simulink model "REXduino_masks"  (Simulink 3.00)
settings: Solver=ode45  SolverMode=SingleTasking  StartTime=0.0  StopTime=10.0  RelTol=1e-3
libraries: logiclib x194, mathlib x116, analoglib x15, genlib x12, speclib x4
(part 1 of 2)
settings Model: ExtModeTrigMode=normal  ExtModeArmWhenConnect=on  Creator=jsobota  LastModifiedBy=XPMUser

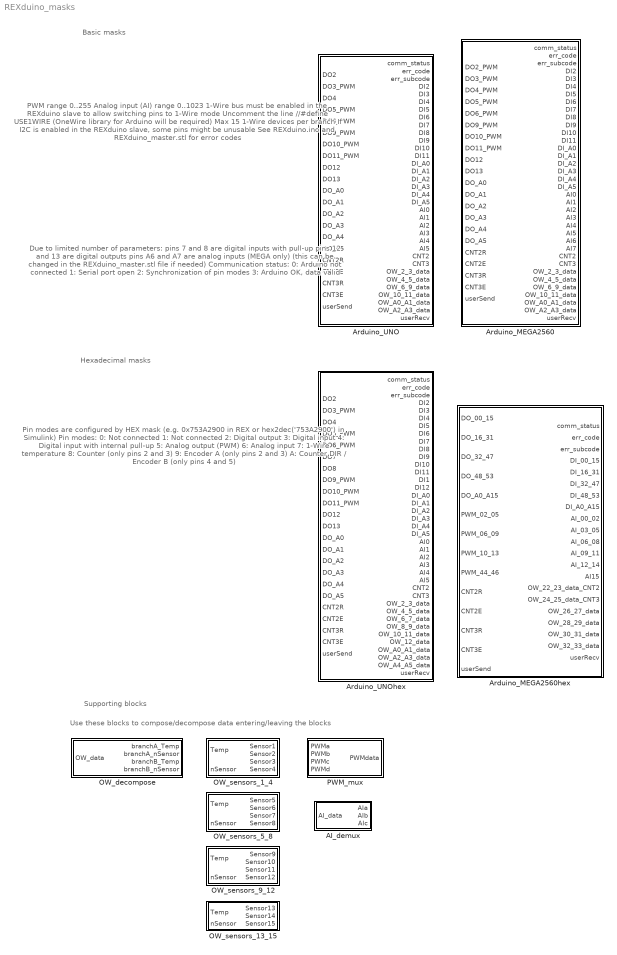
== system REXduino_masks ==
  note: Basic masks
  note: PWM range 0..255
      |
      | Analog input (AI) range 0..1023
      |
      | 1-Wire bus must be enabled in the REXduino slave
      | to allow switching pins to 1-Wire mode
      | Uncomment the line //#define USE1WIRE
      | (OneWire library for Arduino will be required)
      |
      | Max 15 1-Wire devices per branch
      |
      | If I2C is enabled in the REXduino slave, some pins
      | might be unusable
      |
      | See REXduino.ino and REXduino_master.stl for error codes
  note: Hexadecimal masks
  note: Pin modes are configured by HEX mask
      |    (e.g. 0x753A2900 in REX or hex2dec('753A2900') in Simulink)
      |
      | Pin modes:
      | 0: Not connected
      | 1: Not connected
      | 2: Digital output
      | 3: Digital input
      | 4: Digital input with internal pull-up
      | 5: Analog output (PWM)
      | 6: Analog input
      | 7: 1-Wire temperature
      | 8: Counter (only pins 2 and 3)
      | 9: Encoder A (only pins 2 and 3)
      | A: Counter DIR / Encoder B (only pins 4 and 5)
  note: Supporting blocks
  note: Use these blocks to compose/decompose data entering/leaving the blocks
  note: Due to limited number of parameters:
      | pins 7 and 8 are digital inputs with pull-up
      | pins 12 and 13 are digital outputs
      | pins A6 and A7 are analog inputs (MEGA only)
      | (this can be changed in the REXduino_master.stl file if needed)
      |
      | Communication status:
      | 0: Arduino not connected
      | 1: Serial port open
      | 2: Synchronization of pin modes
      | 3: Arduino OK, data valid
  AI_demux : Subsystem
      mask Type: REX sequence
  Arduino_MEGA2560 : Subsystem  mask(REX sequence){comPort=/dev/ttyACM0, pinmode2=1: Not connected, pinmode3=1: Not connected, pinmode4=1: Not connected, pinmode5=1: Not connected, pinmode6=1: Not connected, pinmode9=1: Not connected, pinmode10=1: Not connected, pinmode11=1: Not connected, pinmodeA0=1: Not connected, pinmodeA1=1: Not connected, pinmodeA2=1: Not connected, pinmodeA3=1: Not connected, pinmodeA4=1: Not connected, pinmodeA5=1: Not connected}
      mask prompts: comPort "Serial device, e.g. COM7, /dev/ttyACM0, /dev/ttyUSB0 etc."; pinmode2 "Pin 2 mode"; pinmode3 "Pin 2 mode"; pinmode4 "Pin 2 mode"; pinmode5 "Pin 2 mode"; pinmode6 "Pin 2 mode"; pinmode9 "Pin 2 mode"; pinmode10 "Pin 2 mode"; pinmode11 "Pin 2 mode"; pinmodeA0 "Pin 2 mode"; pinmodeA1 "Pin 2 mode"; pinmodeA2 "Pin 2 mode"; pinmodeA3 "Pin 2 mode"; pinmodeA4 "Pin 2 mode"; pinmodeA5 "Pin 2 mode"
      mask StyleString: edit,popup(1: Not connected|2: Digital output|3: Digital input|4: Digital input with internal pull-up|5: PWM (analog output)|6: --- N/A for this pin ---|7: 1-Wire temperature|8: Counter|9: Encoder),popup(1: Not connected|2: Digital output|3: Digital input|4: Digital input with internal pull-up|5: PWM (analog output)|6: --- N/A for this pin ---|7: 1-Wire temperature|8: Counter|9: Encoder),popup(1: Not connected|2: Digital output|3: Digital input|4: Digital input with internal pull-up|5: PWM (analog output)|6: --- N/A for this pin ---|7: 1-Wire temperature|8: --- N/A for this pin ---|9: --- N/A for this pin ---|10: Counter DIR / Encoder B),popup(1: Not connected|2: Digital output|3: Digital input|4: Digital input with internal pull-up|5: PWM (analog output)|6: --- N/A for this pin ---|7: 1-Wire temperature|8: --- N/A for this pin ---|9: --- N/A for this pin ---|10: Counter DIR / Encoder B),popup(1: Not connected|2: Digital output|3: Digital input|4: Digital input with internal pull-up|5: PWM (analog output)|6: --- N/A for this pin ---|7: 1-Wire temperature),popup(1: Not connected|2: Digital output|3: Digital input|4: Digital input with internal pull-up|5: PWM (analog output)|6: --- N/A for this pin ---|7: 1-Wire temperature),popup(1: Not connected|2: Digital output|3: Digital input|4: Digital input with internal pull-up|5: PWM (analog output)|6: --- N/A for this pin ---|7: 1-Wire temperature),popup(1: Not connected|2: Digital output|3: Digital input|4: Digital input with internal pull-up|5: PWM (analog output)|6: --- N/A for this pin|7: 1-Wire temperature),popup(1: Not connected|2: Digital output|3: Digital input|4: Digital input with internal pull-up|5: --- N/A for this pin ---|6: Analog input|7: 1-Wire temperature),popup(1: Not connected|2: Digital output|3: Digital input|4: Digital input with internal pull-up|5: --- N/A for this pin ---|6: Analog input|7: 1-Wire temperature),popup(1: Not connected|2: Digital output|3: Digital input|4: Digital input with internal pull-up|5: --- N/A for this pin ---|6: Analog input|7: 1-Wire temperature),popup(1: Not connected|2: Digital output|3: Digital input|4: Digital input with internal pull-up|5: --- N/A for this pin ---|6: Analog input|7: 1-Wire temperature),popup(1: Not connected|2: Digital output|3: Digital input|4: Digital input with internal pull-up|5: --- N/A for this pin ---|6: Analog input|7: 1-Wire temperature),popup(1: Not connected|2: Digital output|3: Digital input|4: Digital input with internal pull-up|5: --- N/A for this pin ---|6: Analog input|7: 1-Wire temperature)
      mask CallbackString:
      | REXduino_mask_comPortNo = get_param(gcb,'comPort');
      | REXduino_mask_comPortNo = sscanf(fliplr(REXduino_mask_comPortNo),'%u',1);
      | if ( ~isempty(REXduino_mask_comPortNo) & (REXduino_mask_comPortNo<100) )
      | set_param([gcb '/CNI_comPortNo'],'icn',fliplr(num2str(REXduino_mask_comPortNo)))
      | else
      | set_param([gcb '/CNI_comPortNo'],'icn','15')
      | end
      | clear REXduino_mask_comPortNo||||||||||||||
  Arduino_MEGA2560hex : Subsystem  mask(REX sequence){comPort=/dev/ttyACM0, pinmodes_00_07=0, pinmodes_08_15=0, pinmodes_16_23=0, pinmodes_24_31=0, pinmodes_32_39=0, pinmodes_40_47=0, pinmodes_48_53=0, pinmodes_A0_A7=0, pinmodes_A8_A15=0}
      mask prompts: comPort "Serial device, e.g. COM7, /dev/ttyACM0, /dev/ttyUSB0 etc."; pinmodes_00_07 "Pin modes 0 to 7 (0 and 1 ignored)"; pinmodes_08_15 "Pin modes 8 to 15"; pinmodes_16_23 "Pin modes 16 to 23"; pinmodes_24_31 "Pin modes 24 to 31"; pinmodes_32_39 "Pin modes 32 to 39"; pinmodes_40_47 "Pin modes 40 to 47"; pinmodes_48_53 "Pin modes 48 to 53"; pinmodes_A0_A7 "Pin modes A0 to A7"; pinmodes_A8_A15 "Pin modes A8 to A15"
      mask CallbackString:
      | REXduino_mask_comPortNo = get_param(gcb,'comPort');
      | REXduino_mask_comPortNo = sscanf(fliplr(REXduino_mask_comPortNo),'%u',1);
      | if ( ~isempty(REXduino_mask_comPortNo) & (REXduino_mask_comPortNo<100) )
      | set_param([gcb '/CNI_comPortNo'],'icn',fliplr(num2str(REXduino_mask_comPortNo)))
      | else
      | set_param([gcb '/CNI_comPortNo'],'icn','15')
      | end
      | clear REXduino_mask_comPortNo|||||||||
  Arduino_UNO : Subsystem  mask(REX sequence){comPort=/dev/ttyACM0, pinmode2=1: Not connected, pinmode3=1: Not connected, pinmode4=1: Not connected, pinmode5=1: Not connected, pinmode6=1: Not connected, pinmode9=1: Not connected, pinmode10=1: Not connected, pinmode11=1: Not connected, pinmodeA0=1: Not connected, pinmodeA1=1: Not connected, pinmodeA2=1: Not connected, pinmodeA3=1: Not connected, pinmodeA4=1: Not connected, pinmodeA5=1: Not connected}
      mask prompts: comPort "Serial device, e.g. COM7, /dev/ttyACM0, /dev/ttyUSB0 etc."; pinmode2 "Pin 2 mode"; pinmode3 "Pin 2 mode"; pinmode4 "Pin 2 mode"; pinmode5 "Pin 2 mode"; pinmode6 "Pin 2 mode"; pinmode9 "Pin 2 mode"; pinmode10 "Pin 2 mode"; pinmode11 "Pin 2 mode"; pinmodeA0 "Pin 2 mode"; pinmodeA1 "Pin 2 mode"; pinmodeA2 "Pin 2 mode"; pinmodeA3 "Pin 2 mode"; pinmodeA4 "Pin 2 mode"; pinmodeA5 "Pin 2 mode"
      mask StyleString: edit,popup(1: Not connected|2: Digital output|3: Digital input|4: Digital input with internal pull-up|5: --- N/A for this pin ---|6: --- N/A for this pin ---|7: 1-Wire temperature|8: Counter|9: Encoder A),popup(1: Not connected|2: Digital output|3: Digital input|4: Digital input with internal pull-up|5: PWM (analog output)|6: --- N/A for this pin ---|7: 1-Wire temperature|8: Counter|9: Encoder A),popup(1: Not connected|2: Digital output|3: Digital input|4: Digital input with internal pull-up|5: --- N/A for this pin ---|6: --- N/A for this pin ---|7: 1-Wire temperature|8: --- N/A for this pin ---|9: --- N/A for this pin ---|10: Counter DIR / Encoder B),popup(1: Not connected|2: Digital output|3: Digital input|4: Digital input with internal pull-up|5: PWM (analog output)|6: --- N/A for this pin ---|7: 1-Wire temperature|8: --- N/A for this pin ---|9: --- N/A for this pin ---|10: Counter DIR / Encoder B),popup(1: Not connected|2: Digital output|3: Digital input|4: Digital input with internal pull-up|5: PWM (analog output)|6: --- N/A for this pin ---|7: 1-Wire temperature),popup(1: Not connected|2: Digital output|3: Digital input|4: Digital input with internal pull-up|5: PWM (analog output)|6: --- N/A for this pin ---|7: 1-Wire temperature),popup(1: Not connected|2: Digital output|3: Digital input|4: Digital input with internal pull-up|5: PWM (analog output)|6: --- N/A for this pin ---|7: 1-Wire temperature),popup(1: Not connected|2: Digital output|3: Digital input|4: Digital input with internal pull-up|5: PWM (analog output)|6: --- N/A for this pin ---|7: 1-Wire temperature),popup(1: Not connected|2: Digital output|3: Digital input|4: Digital input with internal pull-up|5: --- N/A for this pin ---|6: Analog input|7: 1-Wire temperature),popup(1: Not connected|2: Digital output|3: Digital input|4: Digital input with internal pull-up|5: --- N/A for this pin ---|6: Analog input|7: 1-Wire temperature),popup(1: Not connected|2: Digital output|3: Digital input|4: Digital input with internal pull-up|5: --- N/A for this pin ---|6: Analog input|7: 1-Wire temperature),popup(1: Not connected|2: Digital output|3: Digital input|4: Digital input with internal pull-up|5: --- N/A for this pin ---|6: Analog input|7: 1-Wire temperature),popup(1: Not connected|2: Digital output|3: Digital input|4: Digital input with internal pull-up|5: --- N/A for this pin ---|6: Analog input|7: 1-Wire temperature),popup(1: Not connected|2: Digital output|3: Digital input|4: Digital input with internal pull-up|5: --- N/A for this pin ---|6: Analog input|7: 1-Wire temperature)
      mask CallbackString:
      | REXduino_mask_comPortNo = get_param(gcb,'comPort');
      | REXduino_mask_comPortNo = sscanf(fliplr(REXduino_mask_comPortNo),'%u',1);
      | if ( ~isempty(REXduino_mask_comPortNo) & (REXduino_mask_comPortNo<100) )
      | set_param([gcb '/CNI_comPortNo'],'icn',fliplr(num2str(REXduino_mask_comPortNo)))
      | else
      | set_param([gcb '/CNI_comPortNo'],'icn','15')
      | end
      | clear REXduino_mask_comPortNo||||||||||||||
  Arduino_UNOhex : Subsystem  mask(REX sequence){comPort=/dev/ttyACM0, pinmodes_00_07=0, pinmodes_08_13=0, pinmodes_A0_A5=0}
      mask prompts: comPort "Serial device, e.g. COM7, /dev/ttyACM0, /dev/ttyUSB0 etc."; pinmodes_00_07 "Pin modes 0 to 7 (0 and 1 ignored)"; pinmodes_08_13 "Pin modes 8 to 13"; pinmodes_A0_A5 "Pin modes A0 to A5"
      mask CallbackString:
      | REXduino_mask_comPortNo = get_param(gcb,'comPort');
      | REXduino_mask_comPortNo = sscanf(fliplr(REXduino_mask_comPortNo),'%u',1);
      | if ( ~isempty(REXduino_mask_comPortNo) & (REXduino_mask_comPortNo<100) )
      | set_param([gcb '/CNI_comPortNo'],'icn',fliplr(num2str(REXduino_mask_comPortNo)))
      | else
      | set_param([gcb '/CNI_comPortNo'],'icn','15')
      | end
      | clear REXduino_mask_comPortNo|||
  OW_decompose : Subsystem
      mask Type: REX sequence
  OW_sensors_13_15 : Subsystem
      mask Type: REX sequence
  OW_sensors_1_4 : Subsystem
      mask Type: REX sequence
  OW_sensors_5_8 : Subsystem
      mask Type: REX sequence
  OW_sensors_9_12 : Subsystem
      mask Type: REX sequence
  PWM_mux : Subsystem
      mask Type: REX sequence

== system REXduino_masks/AI_demux ==
  AI_data : Inport  Port=1  PortWidth=-1  SampleTime=-1  DataType=auto
      settings: SignalType=auto
  BITOP_1 : logiclib/BITOP  iop=6: Shift Right
  BITOP_10 : logiclib/BITOP  iop=3: Bit AND
  BITOP_2 : logiclib/BITOP  iop=3: Bit AND
  BITOP_3 : logiclib/BITOP  iop=6: Shift Right
  BITOP_4 : logiclib/BITOP  iop=3: Bit AND
  CNI : mathlib/CNI  icn=1023
  CNI_1 : mathlib/CNI  icn=10
  AIa : Outport  Port=1
  AIb : Outport  Port=2
  AIc : Outport  Port=3
  wires:
  AI_data/1 -> BITOP_1/1, BITOP_10/1
  BITOP_1/1 -> BITOP_2/1, BITOP_3/1
  BITOP_10/1 -> AIa/1
  BITOP_2/1 -> AIb/1
  BITOP_3/1 -> BITOP_4/1
  BITOP_4/1 -> AIc/1
  CNI/1 -> BITOP_10/2, BITOP_2/2, BITOP_4/2
  CNI_1/1 -> BITOP_1/2, BITOP_3/2

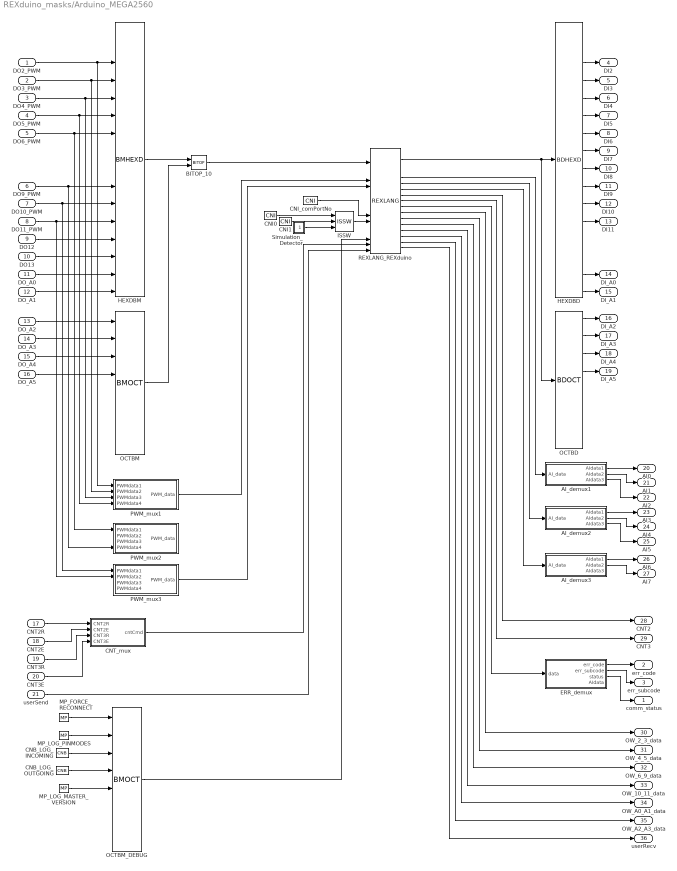
== system REXduino_masks/Arduino_MEGA2560 ==
  DO2_PWM : Inport  Port=1  PortWidth=-1  SampleTime=-1  DataType=auto
      settings: SignalType=auto
  DO3_PWM : Inport  Port=2  PortWidth=-1  SampleTime=-1  DataType=auto
      settings: SignalType=auto
  DO4_PWM : Inport  Port=3  PortWidth=-1  SampleTime=-1  DataType=auto
      settings: SignalType=auto
  DO5_PWM : Inport  Port=4  PortWidth=-1  SampleTime=-1  DataType=auto
      settings: SignalType=auto
  DO6_PWM : Inport  Port=5  PortWidth=-1  SampleTime=-1  DataType=auto
      settings: SignalType=auto
  DO9_PWM : Inport  Port=6  PortWidth=-1  SampleTime=-1  DataType=auto
      settings: SignalType=auto
  DO10_PWM : Inport  Port=7  PortWidth=-1  SampleTime=-1  DataType=auto
      settings: SignalType=auto
  DO11_PWM : Inport  Port=8  PortWidth=-1  SampleTime=-1  DataType=auto
      settings: SignalType=auto
  DO12 : Inport  Port=9  PortWidth=-1  SampleTime=-1  DataType=auto
      settings: SignalType=auto
  DO13 : Inport  Port=10  PortWidth=-1  SampleTime=-1  DataType=auto
      settings: SignalType=auto
  DO_A0 : Inport  Port=11  PortWidth=-1  SampleTime=-1  DataType=auto
      settings: SignalType=auto
  DO_A1 : Inport  Port=12  PortWidth=-1  SampleTime=-1  DataType=auto
      settings: SignalType=auto
  DO_A2 : Inport  Port=13  PortWidth=-1  SampleTime=-1  DataType=auto
      settings: SignalType=auto
  DO_A3 : Inport  Port=14  PortWidth=-1  SampleTime=-1  DataType=auto
      settings: SignalType=auto
  DO_A4 : Inport  Port=15  PortWidth=-1  SampleTime=-1  DataType=auto
      settings: SignalType=auto
  DO_A5 : Inport  Port=16  PortWidth=-1  SampleTime=-1  DataType=auto
      settings: SignalType=auto
  CNT2R : Inport  Port=17  PortWidth=-1  SampleTime=-1  DataType=auto
      settings: SignalType=auto
  CNT2E : Inport  Port=18  PortWidth=-1  SampleTime=-1  DataType=auto
      settings: SignalType=auto
  CNT3R : Inport  Port=19  PortWidth=-1  SampleTime=-1  DataType=auto
      settings: SignalType=auto
  CNT3E : Inport  Port=20  PortWidth=-1  SampleTime=-1  DataType=auto
      settings: SignalType=auto
  userSend : Inport  Port=21  PortWidth=-1  SampleTime=-1  DataType=auto
      settings: SignalType=auto
  AI_demux1 : Subsystem
      mask Type: REX sequence
  AI_demux2 : Subsystem
      mask Type: REX sequence
  AI_demux3 : Subsystem
      mask Type: REX sequence
  BITOP_10 : logiclib/BITOP  iop=2: Bit OR
  CNB_LOG_INCOMING : mathlib/CNB  YCN=off
  CNB_LOG_OUTGOING : mathlib/CNB  YCN=off
  CNI0 : mathlib/CNI  icn=0
  CNI1 : mathlib/CNI  icn=1
  CNI_comPortNo : mathlib/CNI  icn=15
  CNT_mux : Subsystem
      mask Type: REX sequence
  ERR_demux : Subsystem
      mask Type: REX sequence
  HEXDBD : logiclib/BDHEXD  shift=0
  HEXDBM : logiclib/BMHEXD  shift=0
  ISSW : logiclib/ISSW
  MP_FORCE_RECONNECT : genlib/MP  pwidth=10  BSTATE=off  RPTF=off
  MP_LOG_MASTER_VERSION : genlib/MP  pwidth=10  BSTATE=off  RPTF=off
  MP_LOG_PINMODES : genlib/MP  pwidth=10  BSTATE=off  RPTF=off
  OCTBD : logiclib/BDOCT  shift=16
  OCTBM : logiclib/BMOCT  shift=16
  OCTBM_DEBUG : logiclib/BMOCT  shift=0
  PWM_mux1 : Subsystem
      mask Type: REX sequence
  PWM_mux2 : Subsystem
      mask Type: REX sequence
  PWM_mux3 : Subsystem
      mask Type: REX sequence
  REXLANG_REXduino : speclib/REXLANG  strs=0  tab_matlab=MORE  srcname=REXduino_master.c  srctype=1: C-like  stack=0  debug=1: No check  p0=comPort  p1=pinmode2  p2=pinmode3  p3=pinmode4  p4=pinmode5  p5=pinmode6  p6=pinmode9  p7=pinmode10  p8=pinmode11  p9=pinmodeA0  p10=pinmodeA1  p11=pinmodeA2  p12=pinmodeA3  p13=pinmodeA4  p14=pinmodeA5  p15=3
  Simulation_Detector : Subsystem
      mask Type: REX sequence
  comm_status : Outport  Port=1
  err_code : Outport  Port=2
  err_subcode : Outport  Port=3
  DI2 : Outport  Port=4
  DI3 : Outport  Port=5
  DI4 : Outport  Port=6
  DI5 : Outport  Port=7
  DI6 : Outport  Port=8
  DI7 : Outport  Port=9
  DI8 : Outport  Port=10
  DI9 : Outport  Port=11
  DI10 : Outport  Port=12
  DI11 : Outport  Port=13
  DI_A0 : Outport  Port=14
  DI_A1 : Outport  Port=15
  DI_A2 : Outport  Port=16
  DI_A3 : Outport  Port=17
  DI_A4 : Outport  Port=18
  DI_A5 : Outport  Port=19
  AI0 : Outport  Port=20
  AI1 : Outport  Port=21
  AI2 : Outport  Port=22
  AI3 : Outport  Port=23
  AI4 : Outport  Port=24
  AI5 : Outport  Port=25
  AI6 : Outport  Port=26
  AI7 : Outport  Port=27
  CNT2 : Outport  Port=28
  CNT3 : Outport  Port=29
  OW_2_3_data : Outport  Port=30
  OW_4_5_data : Outport  Port=31
  OW_6_9_data : Outport  Port=32
  OW_10_11_data : Outport  Port=33
  OW_A0_A1_data : Outport  Port=34
  OW_A2_A3_data : Outport  Port=35
  userRecv : Outport  Port=36
  wires:
  AI_demux1/1(AIdata1) -> AI0/1
  AI_demux1/2(AIdata2) -> AI1/1
  AI_demux1/3(AIdata3) -> AI2/1
  AI_demux2/1(AIdata1) -> AI3/1
  AI_demux2/2(AIdata2) -> AI4/1
  AI_demux2/3(AIdata3) -> AI5/1
  AI_demux3/1(AIdata1) -> AI6/1
  AI_demux3/2(AIdata2) -> AI7/1
  BITOP_10/1 -> REXLANG_REXduino/3
  CNB_LOG_INCOMING/1 -> OCTBM_DEBUG/3
  CNB_LOG_OUTGOING/1 -> OCTBM_DEBUG/4
  CNI0/1 -> ISSW/1
  CNI1/1 -> ISSW/2
  CNI_comPortNo/1 -> REXLANG_REXduino/12
  CNT2E/1 -> CNT_mux/2(CNT2E)
  CNT2R/1 -> CNT_mux/1(CNT2R)
  CNT3E/1 -> CNT_mux/4(CNT3E)
  CNT3R/1 -> CNT_mux/3(CNT3R)
  CNT_mux/1(cntCmd) -> REXLANG_REXduino/17
  DO10_PWM/1 -> HEXDBM/11, PWM_mux3/1(PWMdata1)
  DO11_PWM/1 -> HEXDBM/12, PWM_mux3/2(PWMdata2)
  DO12/1 -> HEXDBM/13
  DO13/1 -> HEXDBM/14
  DO2_PWM/1 -> HEXDBM/3, PWM_mux1/1(PWMdata1)
  DO3_PWM/1 -> HEXDBM/4, PWM_mux1/2(PWMdata2)
  DO4_PWM/1 -> HEXDBM/5, PWM_mux1/3(PWMdata3)
  DO5_PWM/1 -> HEXDBM/6, PWM_mux1/4(PWMdata4)
  DO6_PWM/1 -> HEXDBM/7, PWM_mux2/1(PWMdata1)
  DO9_PWM/1 -> HEXDBM/10, PWM_mux2/4(PWMdata4)
  DO_A0/1 -> HEXDBM/15
  DO_A1/1 -> HEXDBM/16
  DO_A2/1 -> OCTBM/1
  DO_A3/1 -> OCTBM/2
  DO_A4/1 -> OCTBM/3
  DO_A5/1 -> OCTBM/4
  ERR_demux/1(err_code) -> err_code/1
  ERR_demux/2(err_subcode) -> err_subcode/1
  ERR_demux/3(status) -> comm_status/1
  HEXDBD/3 -> DI2/1
  HEXDBD/4 -> DI3/1
  HEXDBD/5 -> DI4/1
  HEXDBD/6 -> DI5/1
  HEXDBD/7 -> DI6/1
  HEXDBD/8 -> DI7/1
  HEXDBD/9 -> DI8/1
  HEXDBD/10 -> DI9/1
  HEXDBD/11 -> DI10/1
  HEXDBD/12 -> DI11/1
  HEXDBD/15 -> DI_A0/1
  HEXDBD/16 -> DI_A1/1
  HEXDBM/1 -> BITOP_10/1
  ISSW/1 -> REXLANG_REXduino/13
  MP_FORCE_RECONNECT/1 -> OCTBM_DEBUG/1
  MP_LOG_MASTER_VERSION/1 -> OCTBM_DEBUG/5
  MP_LOG_PINMODES/1 -> OCTBM_DEBUG/2
  OCTBD/1 -> DI_A2/1
  OCTBD/2 -> DI_A3/1
  OCTBD/3 -> DI_A4/1
  OCTBD/4 -> DI_A5/1
  OCTBM/1 -> BITOP_10/2
  OCTBM_DEBUG/1 -> REXLANG_REXduino/16
  PWM_mux1/1(PWM_data) -> REXLANG_REXduino/6
  PWM_mux3/1(PWM_data) -> REXLANG_REXduino/7
  REXLANG_REXduino/2 -> HEXDBD/1, OCTBD/1
  REXLANG_REXduino/5 -> AI_demux1/1(AI_data)
  REXLANG_REXduino/6 -> AI_demux2/1(AI_data)
  REXLANG_REXduino/7 -> AI_demux3/1(AI_data)
  REXLANG_REXduino/8 -> CNT2/1
  REXLANG_REXduino/9 -> CNT3/1
  REXLANG_REXduino/10 -> ERR_demux/1(data)
  REXLANG_REXduino/11 -> OW_2_3_data/1
  REXLANG_REXduino/12 -> OW_4_5_data/1
  REXLANG_REXduino/13 -> OW_6_9_data/1
  REXLANG_REXduino/14 -> OW_10_11_data/1
  REXLANG_REXduino/15 -> OW_A0_A1_data/1
  REXLANG_REXduino/16 -> OW_A2_A3_data/1
  REXLANG_REXduino/17 -> userRecv/1
  Simulation_Detector/1(Y) -> ISSW/3
  userSend/1 -> REXLANG_REXduino/18

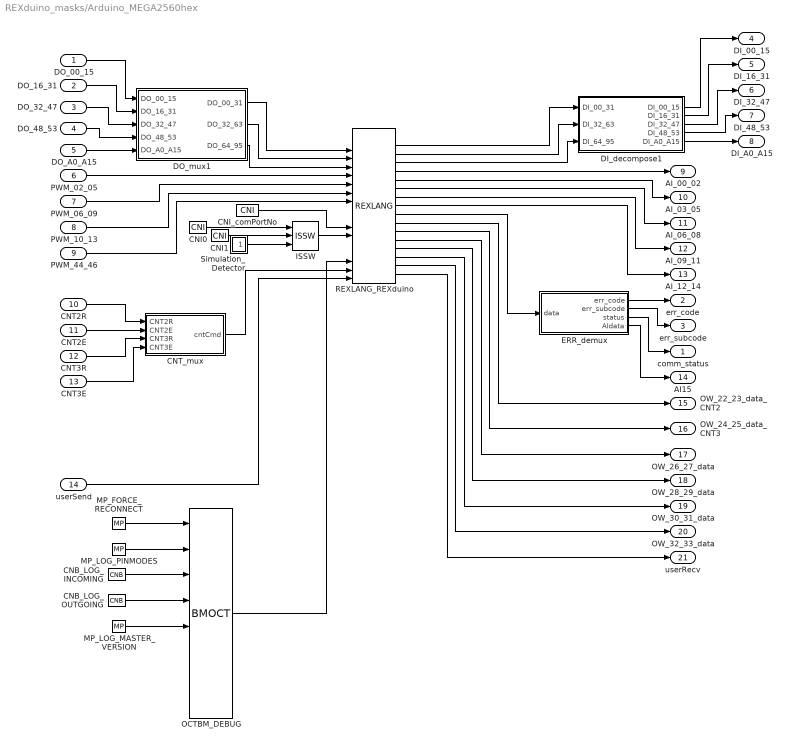
== system REXduino_masks/Arduino_MEGA2560hex ==
  DO_00_15 : Inport  Port=1  PortWidth=-1  SampleTime=-1  DataType=auto
      settings: SignalType=auto
  DO_16_31 : Inport  Port=2  PortWidth=-1  SampleTime=-1  DataType=auto
      settings: SignalType=auto
  DO_32_47 : Inport  Port=3  PortWidth=-1  SampleTime=-1  DataType=auto
      settings: SignalType=auto
  DO_48_53 : Inport  Port=4  PortWidth=-1  SampleTime=-1  DataType=auto
      settings: SignalType=auto
  DO_A0_A15 : Inport  Port=5  PortWidth=-1  SampleTime=-1  DataType=auto
      settings: SignalType=auto
  PWM_02_05 : Inport  Port=6  PortWidth=-1  SampleTime=-1  DataType=auto
      settings: SignalType=auto
  PWM_06_09 : Inport  Port=7  PortWidth=-1  SampleTime=-1  DataType=auto
      settings: SignalType=auto
  PWM_10_13 : Inport  Port=8  PortWidth=-1  SampleTime=-1  DataType=auto
      settings: SignalType=auto
  PWM_44_46 : Inport  Port=9  PortWidth=-1  SampleTime=-1  DataType=auto
      settings: SignalType=auto
  CNT2R : Inport  Port=10  PortWidth=-1  SampleTime=-1  DataType=auto
      settings: SignalType=auto
  CNT2E : Inport  Port=11  PortWidth=-1  SampleTime=-1  DataType=auto
      settings: SignalType=auto
  CNT3R : Inport  Port=12  PortWidth=-1  SampleTime=-1  DataType=auto
      settings: SignalType=auto
  CNT3E : Inport  Port=13  PortWidth=-1  SampleTime=-1  DataType=auto
      settings: SignalType=auto
  userSend : Inport  Port=14  PortWidth=-1  SampleTime=-1  DataType=auto
      settings: SignalType=auto
  CNB_LOG_INCOMING : mathlib/CNB  YCN=off
  CNB_LOG_OUTGOING : mathlib/CNB  YCN=off
  CNI0 : mathlib/CNI  icn=0
  CNI1 : mathlib/CNI  icn=1
  CNI_comPortNo : mathlib/CNI  icn=15
  CNT_mux : Subsystem
      mask Type: REX sequence
  DI_decompose1 : Subsystem
      mask Type: REX sequence
  DO_mux1 : Subsystem
      mask Type: REX sequence
  ERR_demux : Subsystem
      mask Type: REX sequence
  ISSW : logiclib/ISSW
  MP_FORCE_RECONNECT : genlib/MP  pwidth=10  BSTATE=off  RPTF=off
  MP_LOG_MASTER_VERSION : genlib/MP  pwidth=10  BSTATE=off  RPTF=off
  MP_LOG_PINMODES : genlib/MP  pwidth=10  BSTATE=off  RPTF=off
  OCTBM_DEBUG : logiclib/BMOCT  shift=0
  REXLANG_REXduino : speclib/REXLANG  strs=0  tab_matlab=MORE  srcname=REXduino_master.c  srctype=1: C-like  stack=0  debug=1: No check  p0=comPort  p1=pinmodes_00_07  p2=pinmodes_08_15  p3=pinmodes_16_23  p4=pinmodes_24_31  p5=pinmodes_32_39  p6=pinmodes_40_47  p7=pinmodes_48_53  p8=pinmodes_A0_A7  p9=pinmodes_A8_A15  p10=0  p11=0  p12=0  p13=0  p14=0  p15=4
  Simulation_Detector : Subsystem
      mask Type: REX sequence
  comm_status : Outport  Port=1
  err_code : Outport  Port=2
  err_subcode : Outport  Port=3
  DI_00_15 : Outport  Port=4
  DI_16_31 : Outport  Port=5
  DI_32_47 : Outport  Port=6
  DI_48_53 : Outport  Port=7
  DI_A0_A15 : Outport  Port=8
  AI_00_02 : Outport  Port=9
  AI_03_05 : Outport  Port=10
  AI_06_08 : Outport  Port=11
  AI_09_11 : Outport  Port=12
  AI_12_14 : Outport  Port=13
  AI15 : Outport  Port=14
  OW_22_23_data_CNT2 : Outport  Port=15
  OW_24_25_data_CNT3 : Outport  Port=16
  OW_26_27_data : Outport  Port=17
  OW_28_29_data : Outport  Port=18
  OW_30_31_data : Outport  Port=19
  OW_32_33_data : Outport  Port=20
  userRecv : Outport  Port=21
  wires:
  CNB_LOG_INCOMING/1 -> OCTBM_DEBUG/3
  CNB_LOG_OUTGOING/1 -> OCTBM_DEBUG/4
  CNI0/1 -> ISSW/1
  CNI1/1 -> ISSW/2
  CNI_comPortNo/1 -> REXLANG_REXduino/12
  CNT2E/1 -> CNT_mux/2(CNT2E)
  CNT2R/1 -> CNT_mux/1(CNT2R)
  CNT3E/1 -> CNT_mux/4(CNT3E)
  CNT3R/1 -> CNT_mux/3(CNT3R)
  CNT_mux/1(cntCmd) -> REXLANG_REXduino/17
  DI_decompose1/1(DI_00_15) -> DI_00_15/1
  DI_decompose1/2(DI_16_31) -> DI_16_31/1
  DI_decompose1/3(DI_32_47) -> DI_32_47/1
  DI_decompose1/4(DI_48_53) -> DI_48_53/1
  DI_decompose1/5(DI_A0_A15) -> DI_A0_A15/1
  DO_00_15/1 -> DO_mux1/1(DO_00_15)
  DO_16_31/1 -> DO_mux1/2(DO_16_31)
  DO_32_47/1 -> DO_mux1/3(DO_32_47)
  DO_48_53/1 -> DO_mux1/4(DO_48_53)
  DO_A0_A15/1 -> DO_mux1/5(DO_A0_A15)
  DO_mux1/1(DO_00_31) -> REXLANG_REXduino/3
  DO_mux1/2(DO_32_63) -> REXLANG_REXduino/4
  DO_mux1/3(DO_64_95) -> REXLANG_REXduino/5
  ERR_demux/1(err_code) -> err_code/1
  ERR_demux/2(err_subcode) -> err_subcode/1
  ERR_demux/3(status) -> comm_status/1
  ERR_demux/4(AIdata) -> AI15/1
  ISSW/1 -> REXLANG_REXduino/13
  MP_FORCE_RECONNECT/1 -> OCTBM_DEBUG/1
  MP_LOG_MASTER_VERSION/1 -> OCTBM_DEBUG/5
  MP_LOG_PINMODES/1 -> OCTBM_DEBUG/2
  OCTBM_DEBUG/1 -> REXLANG_REXduino/16
  PWM_02_05/1 -> REXLANG_REXduino/6
  PWM_06_09/1 -> REXLANG_REXduino/7
  PWM_10_13/1 -> REXLANG_REXduino/8
  PWM_44_46/1 -> REXLANG_REXduino/9
  REXLANG_REXduino/2 -> DI_decompose1/1(DI_00_31)
  REXLANG_REXduino/3 -> DI_decompose1/2(DI_32_63)
  REXLANG_REXduino/4 -> DI_decompose1/3(DI_64_95)
  REXLANG_REXduino/5 -> AI_00_02/1
  REXLANG_REXduino/6 -> AI_03_05/1
  REXLANG_REXduino/7 -> AI_06_08/1
  REXLANG_REXduino/8 -> AI_09_11/1
  REXLANG_REXduino/9 -> AI_12_14/1
  REXLANG_REXduino/10 -> ERR_demux/1(data)
  REXLANG_REXduino/11 -> OW_22_23_data_CNT2/1
  REXLANG_REXduino/12 -> OW_24_25_data_CNT3/1
  REXLANG_REXduino/13 -> OW_26_27_data/1
  REXLANG_REXduino/14 -> OW_28_29_data/1
  REXLANG_REXduino/15 -> OW_30_31_data/1
  REXLANG_REXduino/16 -> OW_32_33_data/1
  REXLANG_REXduino/17 -> userRecv/1
  Simulation_Detector/1(Y) -> ISSW/3
  userSend/1 -> REXLANG_REXduino/18

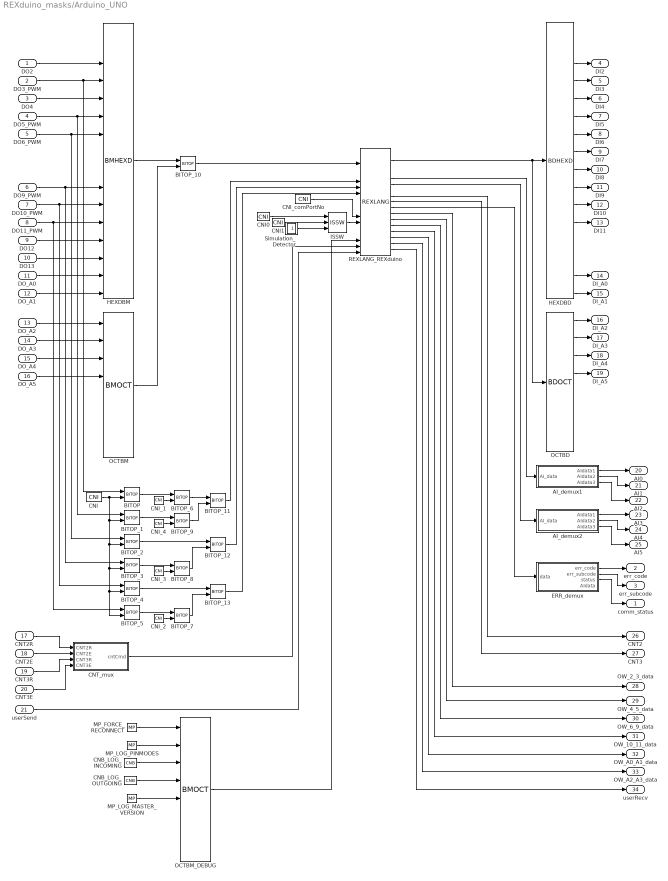
== system REXduino_masks/Arduino_UNO ==
  DO2 : Inport  Port=1  PortWidth=-1  SampleTime=-1  DataType=auto
      settings: SignalType=auto
  DO3_PWM : Inport  Port=2  PortWidth=-1  SampleTime=-1  DataType=auto
      settings: SignalType=auto
  DO4 : Inport  Port=3  PortWidth=-1  SampleTime=-1  DataType=auto
      settings: SignalType=auto
  DO5_PWM : Inport  Port=4  PortWidth=-1  SampleTime=-1  DataType=auto
      settings: SignalType=auto
  DO6_PWM : Inport  Port=5  PortWidth=-1  SampleTime=-1  DataType=auto
      settings: SignalType=auto
  DO9_PWM : Inport  Port=6  PortWidth=-1  SampleTime=-1  DataType=auto
      settings: SignalType=auto
  DO10_PWM : Inport  Port=7  PortWidth=-1  SampleTime=-1  DataType=auto
      settings: SignalType=auto
  DO11_PWM : Inport  Port=8  PortWidth=-1  SampleTime=-1  DataType=auto
      settings: SignalType=auto
  DO12 : Inport  Port=9  PortWidth=-1  SampleTime=-1  DataType=auto
      settings: SignalType=auto
  DO13 : Inport  Port=10  PortWidth=-1  SampleTime=-1  DataType=auto
      settings: SignalType=auto
  DO_A0 : Inport  Port=11  PortWidth=-1  SampleTime=-1  DataType=auto
      settings: SignalType=auto
  DO_A1 : Inport  Port=12  PortWidth=-1  SampleTime=-1  DataType=auto
      settings: SignalType=auto
  DO_A2 : Inport  Port=13  PortWidth=-1  SampleTime=-1  DataType=auto
      settings: SignalType=auto
  DO_A3 : Inport  Port=14  PortWidth=-1  SampleTime=-1  DataType=auto
      settings: SignalType=auto
  DO_A4 : Inport  Port=15  PortWidth=-1  SampleTime=-1  DataType=auto
      settings: SignalType=auto
  DO_A5 : Inport  Port=16  PortWidth=-1  SampleTime=-1  DataType=auto
      settings: SignalType=auto
  CNT2R : Inport  Port=17  PortWidth=-1  SampleTime=-1  DataType=auto
      settings: SignalType=auto
  CNT2E : Inport  Port=18  PortWidth=-1  SampleTime=-1  DataType=auto
      settings: SignalType=auto
  CNT3R : Inport  Port=19  PortWidth=-1  SampleTime=-1  DataType=auto
      settings: SignalType=auto
  CNT3E : Inport  Port=20  PortWidth=-1  SampleTime=-1  DataType=auto
      settings: SignalType=auto
  userSend : Inport  Port=21  PortWidth=-1  SampleTime=-1  DataType=auto
      settings: SignalType=auto
  AI_demux1 : Subsystem
      mask Type: REX sequence
  AI_demux2 : Subsystem
      mask Type: REX sequence
  BITOP : logiclib/BITOP  iop=3: Bit AND
  BITOP_{1..5} (5 alike) : logiclib/BITOP  iop=3: Bit AND
  BITOP_{10..13} (4 alike) : logiclib/BITOP  iop=2: Bit OR
  BITOP_{6..9} (4 alike) : logiclib/BITOP  iop=5: Shift Left
  CNB_LOG_INCOMING : mathlib/CNB  YCN=off
  CNB_LOG_OUTGOING : mathlib/CNB  YCN=off
  CNI : mathlib/CNI  icn=255
  CNI0 : mathlib/CNI  icn=0
  CNI1 : mathlib/CNI  icn=1
  CNI_1 : mathlib/CNI  icn=8
  CNI_2 : mathlib/CNI  icn=8
  CNI_3 : mathlib/CNI  icn=24
  CNI_4 : mathlib/CNI  icn=24
  CNI_comPortNo : mathlib/CNI  icn=15
  CNT_mux : Subsystem
      mask Type: REX sequence
  ERR_demux : Subsystem
      mask Type: REX sequence
  HEXDBD : logiclib/BDHEXD  shift=0
  HEXDBM : logiclib/BMHEXD  shift=0
  ISSW : logiclib/ISSW
  MP_FORCE_RECONNECT : genlib/MP  pwidth=10  BSTATE=off  RPTF=off
  MP_LOG_MASTER_VERSION : genlib/MP  pwidth=10  BSTATE=off  RPTF=off
  MP_LOG_PINMODES : genlib/MP  pwidth=10  BSTATE=off  RPTF=off
  OCTBD : logiclib/BDOCT  shift=16
  OCTBM : logiclib/BMOCT  shift=16
  OCTBM_DEBUG : logiclib/BMOCT  shift=0
  REXLANG_REXduino : speclib/REXLANG  strs=0  tab_matlab=MORE  srcname=REXduino_master.c  srctype=1: C-like  stack=0  debug=1: No check  p0=comPort  p1=pinmode2  p2=pinmode3  p3=pinmode4  p4=pinmode5  p5=pinmode6  p6=pinmode9  p7=pinmode10  p8=pinmode11  p9=pinmodeA0  p10=pinmodeA1  p11=pinmodeA2  p12=pinmodeA3  p13=pinmodeA4  p14=pinmodeA5  p15=1
  Simulation_Detector : Subsystem
      mask Type: REX sequence
  comm_status : Outport  Port=1
  err_code : Outport  Port=2
  err_subcode : Outport  Port=3
  DI2 : Outport  Port=4
  DI3 : Outport  Port=5
  DI4 : Outport  Port=6
  DI5 : Outport  Port=7
  DI6 : Outport  Port=8
  DI7 : Outport  Port=9
  DI8 : Outport  Port=10
  DI9 : Outport  Port=11
  DI10 : Outport  Port=12
  DI11 : Outport  Port=13
  DI_A0 : Outport  Port=14
  DI_A1 : Outport  Port=15
  DI_A2 : Outport  Port=16
  DI_A3 : Outport  Port=17
  DI_A4 : Outport  Port=18
  DI_A5 : Outport  Port=19
  AI0 : Outport  Port=20
  AI1 : Outport  Port=21
  AI2 : Outport  Port=22
  AI3 : Outport  Port=23
  AI4 : Outport  Port=24
  AI5 : Outport  Port=25
  CNT2 : Outport  Port=26
  CNT3 : Outport  Port=27
  OW_2_3_data : Outport  Port=28
  OW_4_5_data : Outport  Port=29
  OW_6_9_data : Outport  Port=30
  OW_10_11_data : Outport  Port=31
  OW_A0_A1_data : Outport  Port=32
  OW_A2_A3_data : Outport  Port=33
  userRecv : Outport  Port=34
  wires:
  AI_demux1/1(AIdata1) -> AI0/1
  AI_demux1/2(AIdata2) -> AI1/1
  AI_demux1/3(AIdata3) -> AI2/1
  AI_demux2/1(AIdata1) -> AI3/1
  AI_demux2/2(AIdata2) -> AI4/1
  AI_demux2/3(AIdata3) -> AI5/1
  BITOP/1 -> BITOP_6/1
  BITOP_1/1 -> BITOP_9/1
  BITOP_10/1 -> REXLANG_REXduino/3
  BITOP_11/1 -> REXLANG_REXduino/6
  BITOP_12/1 -> REXLANG_REXduino/7
  BITOP_13/1 -> REXLANG_REXduino/8
  BITOP_2/1 -> BITOP_12/1
  BITOP_3/1 -> BITOP_8/1
  BITOP_4/1 -> BITOP_13/1
  BITOP_5/1 -> BITOP_7/1
  BITOP_6/1 -> BITOP_11/1
  BITOP_7/1 -> BITOP_13/2
  BITOP_8/1 -> BITOP_12/2
  BITOP_9/1 -> BITOP_11/2
  CNB_LOG_INCOMING/1 -> OCTBM_DEBUG/3
  CNB_LOG_OUTGOING/1 -> OCTBM_DEBUG/4
  CNI/1 -> BITOP/2, BITOP_1/2, BITOP_2/2, BITOP_3/2, BITOP_4/2, BITOP_5/2
  CNI0/1 -> ISSW/1
  CNI1/1 -> ISSW/2
  CNI_1/1 -> BITOP_6/2
  CNI_2/1 -> BITOP_7/2
  CNI_3/1 -> BITOP_8/2
  CNI_4/1 -> BITOP_9/2
  CNI_comPortNo/1 -> REXLANG_REXduino/12
  CNT2E/1 -> CNT_mux/2(CNT2E)
  CNT2R/1 -> CNT_mux/1(CNT2R)
  CNT3E/1 -> CNT_mux/4(CNT3E)
  CNT3R/1 -> CNT_mux/3(CNT3R)
  CNT_mux/1(cntCmd) -> REXLANG_REXduino/17
  DO10_PWM/1 -> BITOP_4/1, HEXDBM/11
  DO11_PWM/1 -> BITOP_5/1, HEXDBM/12
  DO12/1 -> HEXDBM/13
  DO13/1 -> HEXDBM/14
  DO2/1 -> HEXDBM/3
  DO3_PWM/1 -> BITOP/1, HEXDBM/4
  DO4/1 -> HEXDBM/5
  DO5_PWM/1 -> BITOP_1/1, HEXDBM/6
  DO6_PWM/1 -> BITOP_2/1, HEXDBM/7
  DO9_PWM/1 -> BITOP_3/1, HEXDBM/10
  DO_A0/1 -> HEXDBM/15
  DO_A1/1 -> HEXDBM/16
  DO_A2/1 -> OCTBM/1
  DO_A3/1 -> OCTBM/2
  DO_A4/1 -> OCTBM/3
  DO_A5/1 -> OCTBM/4
  ERR_demux/1(err_code) -> err_code/1
  ERR_demux/2(err_subcode) -> err_subcode/1
  ERR_demux/3(status) -> comm_status/1
  HEXDBD/3 -> DI2/1
  HEXDBD/4 -> DI3/1
  HEXDBD/5 -> DI4/1
  HEXDBD/6 -> DI5/1
  HEXDBD/7 -> DI6/1
  HEXDBD/8 -> DI7/1
  HEXDBD/9 -> DI8/1
  HEXDBD/10 -> DI9/1
  HEXDBD/11 -> DI10/1
  HEXDBD/12 -> DI11/1
  HEXDBD/15 -> DI_A0/1
  HEXDBD/16 -> DI_A1/1
  HEXDBM/1 -> BITOP_10/1
  ISSW/1 -> REXLANG_REXduino/13
  MP_FORCE_RECONNECT/1 -> OCTBM_DEBUG/1
  MP_LOG_MASTER_VERSION/1 -> OCTBM_DEBUG/5
  MP_LOG_PINMODES/1 -> OCTBM_DEBUG/2
  OCTBD/1 -> DI_A2/1
  OCTBD/2 -> DI_A3/1
  OCTBD/3 -> DI_A4/1
  OCTBD/4 -> DI_A5/1
  OCTBM/1 -> BITOP_10/2
  OCTBM_DEBUG/1 -> REXLANG_REXduino/16
  REXLANG_REXduino/2 -> HEXDBD/1, OCTBD/1
  REXLANG_REXduino/5 -> AI_demux1/1(AI_data)
  REXLANG_REXduino/6 -> AI_demux2/1(AI_data)
  REXLANG_REXduino/8 -> CNT2/1
  REXLANG_REXduino/9 -> CNT3/1
  REXLANG_REXduino/10 -> ERR_demux/1(data)
  REXLANG_REXduino/11 -> OW_2_3_data/1
  REXLANG_REXduino/12 -> OW_4_5_data/1
  REXLANG_REXduino/13 -> OW_6_9_data/1
  REXLANG_REXduino/14 -> OW_10_11_data/1
  REXLANG_REXduino/15 -> OW_A0_A1_data/1
  REXLANG_REXduino/16 -> OW_A2_A3_data/1
  REXLANG_REXduino/17 -> userRecv/1
  Simulation_Detector/1(Y) -> ISSW/3
  userSend/1 -> REXLANG_REXduino/18

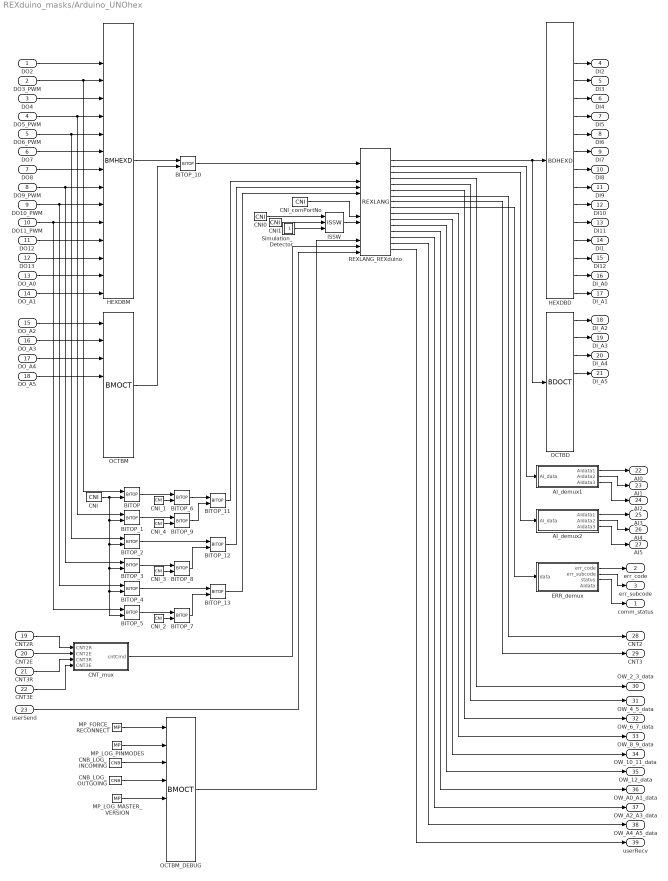
== system REXduino_masks/Arduino_UNOhex ==
  DO2 : Inport  Port=1  PortWidth=-1  SampleTime=-1  DataType=auto
      settings: SignalType=auto
  DO3_PWM : Inport  Port=2  PortWidth=-1  SampleTime=-1  DataType=auto
      settings: SignalType=auto
  DO4 : Inport  Port=3  PortWidth=-1  SampleTime=-1  DataType=auto
      settings: SignalType=auto
  DO5_PWM : Inport  Port=4  PortWidth=-1  SampleTime=-1  DataType=auto
      settings: SignalType=auto
  DO6_PWM : Inport  Port=5  PortWidth=-1  SampleTime=-1  DataType=auto
      settings: SignalType=auto
  DO7 : Inport  Port=6  PortWidth=-1  SampleTime=-1  DataType=auto
      settings: SignalType=auto
  DO8 : Inport  Port=7  PortWidth=-1  SampleTime=-1  DataType=auto
      settings: SignalType=auto
  DO9_PWM : Inport  Port=8  PortWidth=-1  SampleTime=-1  DataType=auto
      settings: SignalType=auto
  DO10_PWM : Inport  Port=9  PortWidth=-1  SampleTime=-1  DataType=auto
      settings: SignalType=auto
  DO11_PWM : Inport  Port=10  PortWidth=-1  SampleTime=-1  DataType=auto
      settings: SignalType=auto
  DO12 : Inport  Port=11  PortWidth=-1  SampleTime=-1  DataType=auto
      settings: SignalType=auto
  DO13 : Inport  Port=12  PortWidth=-1  SampleTime=-1  DataType=auto
      settings: SignalType=auto
  DO_A0 : Inport  Port=13  PortWidth=-1  SampleTime=-1  DataType=auto
      settings: SignalType=auto
  DO_A1 : Inport  Port=14  PortWidth=-1  SampleTime=-1  DataType=auto
      settings: SignalType=auto
  DO_A2 : Inport  Port=15  PortWidth=-1  SampleTime=-1  DataType=auto
      settings: SignalType=auto
  DO_A3 : Inport  Port=16  PortWidth=-1  SampleTime=-1  DataType=auto
      settings: SignalType=auto
  DO_A4 : Inport  Port=17  PortWidth=-1  SampleTime=-1  DataType=auto
      settings: SignalType=auto
  DO_A5 : Inport  Port=18  PortWidth=-1  SampleTime=-1  DataType=auto
      settings: SignalType=auto
  CNT2R : Inport  Port=19  PortWidth=-1  SampleTime=-1  DataType=auto
      settings: SignalType=auto
  CNT2E : Inport  Port=20  PortWidth=-1  SampleTime=-1  DataType=auto
      settings: SignalType=auto
  CNT3R : Inport  Port=21  PortWidth=-1  SampleTime=-1  DataType=auto
      settings: SignalType=auto
  CNT3E : Inport  Port=22  PortWidth=-1  SampleTime=-1  DataType=auto
      settings: SignalType=auto
  userSend : Inport  Port=23  PortWidth=-1  SampleTime=-1  DataType=auto
      settings: SignalType=auto
  AI_demux1 : Subsystem
      mask Type: REX sequence
  AI_demux2 : Subsystem
      mask Type: REX sequence
  BITOP : logiclib/BITOP  iop=3: Bit AND
  BITOP_{1..5} (5 alike) : logiclib/BITOP  iop=3: Bit AND
  BITOP_{10..13} (4 alike) : logiclib/BITOP  iop=2: Bit OR
  BITOP_{6..9} (4 alike) : logiclib/BITOP  iop=5: Shift Left
  CNB_LOG_INCOMING : mathlib/CNB  YCN=off
  CNB_LOG_OUTGOING : mathlib/CNB  YCN=off
  CNI : mathlib/CNI  icn=255
  CNI0 : mathlib/CNI  icn=0
  CNI1 : mathlib/CNI  icn=1
  CNI_1 : mathlib/CNI  icn=8
  CNI_2 : mathlib/CNI  icn=8
  CNI_3 : mathlib/CNI  icn=24
  CNI_4 : mathlib/CNI  icn=24
  CNI_comPortNo : mathlib/CNI  icn=15
  CNT_mux : Subsystem
      mask Type: REX sequence
  ERR_demux : Subsystem
      mask Type: REX sequence
  HEXDBD : logiclib/BDHEXD  shift=0
  HEXDBM : logiclib/BMHEXD  shift=0
  ISSW : logiclib/ISSW
  MP_FORCE_RECONNECT : genlib/MP  pwidth=10  BSTATE=off  RPTF=off
  MP_LOG_MASTER_VERSION : genlib/MP  pwidth=10  BSTATE=off  RPTF=off
  MP_LOG_PINMODES : genlib/MP  pwidth=10  BSTATE=off  RPTF=off
  OCTBD : logiclib/BDOCT  shift=16
  OCTBM : logiclib/BMOCT  shift=16
  OCTBM_DEBUG : logiclib/BMOCT  shift=0
  REXLANG_REXduino : speclib/REXLANG  strs=0  tab_matlab=MORE  srcname=REXduino_master.c  srctype=1: C-like  stack=0  debug=1: No check  p0=comPort  p1=pinmodes_00_07  p2=pinmodes_08_13  p3=pinmodes_A0_A5  p4=0  p5=0  p6=0  p7=0  p8=0  p9=0  p10=0  p11=0  p12=0  p13=0  p14=0  p15=2
  Simulation_Detector : Subsystem
      mask Type: REX sequence
  comm_status : Outport  Port=1
  err_code : Outport  Port=2
  err_subcode : Outport  Port=3
  DI2 : Outport  Port=4
  DI3 : Outport  Port=5
  DI4 : Outport  Port=6
  DI5 : Outport  Port=7
  DI6 : Outport  Port=8
  DI7 : Outport  Port=9
  DI8 : Outport  Port=10
  DI9 : Outport  Port=11
  DI10 : Outport  Port=12
  DI11 : Outport  Port=13
  DI1 : Outport  Port=14
  DI12 : Outport  Port=15
  DI_A0 : Outport  Port=16
  DI_A1 : Outport  Port=17
  DI_A2 : Outport  Port=18
  DI_A3 : Outport  Port=19
  DI_A4 : Outport  Port=20
  DI_A5 : Outport  Port=21
  AI0 : Outport  Port=22
  AI1 : Outport  Port=23
  AI2 : Outport  Port=24
  AI3 : Outport  Port=25
  AI4 : Outport  Port=26
  AI5 : Outport  Port=27
  CNT2 : Outport  Port=28
  CNT3 : Outport  Port=29
  OW_2_3_data : Outport  Port=30
  OW_4_5_data : Outport  Port=31
  OW_6_7_data : Outport  Port=32
  OW_8_9_data : Outport  Port=33
  OW_10_11_data : Outport  Port=34
  OW_12_data : Outport  Port=35
  OW_A0_A1_data : Outport  Port=36
  OW_A2_A3_data : Outport  Port=37
  OW_A4_A5_data : Outport  Port=38
  userRecv : Outport  Port=39
  wires:
  AI_demux1/1(AIdata1) -> AI0/1
  AI_demux1/2(AIdata2) -> AI1/1
  AI_demux1/3(AIdata3) -> AI2/1
  AI_demux2/1(AIdata1) -> AI3/1
  AI_demux2/2(AIdata2) -> AI4/1
  AI_demux2/3(AIdata3) -> AI5/1
  BITOP/1 -> BITOP_6/1
  BITOP_1/1 -> BITOP_9/1
  BITOP_10/1 -> REXLANG_REXduino/3
  BITOP_11/1 -> REXLANG_REXduino/6
  BITOP_12/1 -> REXLANG_REXduino/7
  BITOP_13/1 -> REXLANG_REXduino/8
  BITOP_2/1 -> BITOP_12/1
  BITOP_3/1 -> BITOP_8/1
  BITOP_4/1 -> BITOP_13/1
  BITOP_5/1 -> BITOP_7/1
  BITOP_6/1 -> BITOP_11/1
  BITOP_7/1 -> BITOP_13/2
  BITOP_8/1 -> BITOP_12/2
  BITOP_9/1 -> BITOP_11/2
  CNB_LOG_INCOMING/1 -> OCTBM_DEBUG/3
  CNB_LOG_OUTGOING/1 -> OCTBM_DEBUG/4
  CNI/1 -> BITOP/2, BITOP_1/2, BITOP_2/2, BITOP_3/2, BITOP_4/2, BITOP_5/2
  CNI0/1 -> ISSW/1
  CNI1/1 -> ISSW/2
  CNI_1/1 -> BITOP_6/2
  CNI_2/1 -> BITOP_7/2
  CNI_3/1 -> BITOP_8/2
  CNI_4/1 -> BITOP_9/2
  CNI_comPortNo/1 -> REXLANG_REXduino/12
  CNT2E/1 -> CNT_mux/2(CNT2E)
  CNT2R/1 -> CNT_mux/1(CNT2R)
  CNT3E/1 -> CNT_mux/4(CNT3E)
  CNT3R/1 -> CNT_mux/3(CNT3R)
  CNT_mux/1(cntCmd) -> REXLANG_REXduino/17
  DO10_PWM/1 -> BITOP_4/1, HEXDBM/11
  DO11_PWM/1 -> BITOP_5/1, HEXDBM/12
  DO12/1 -> HEXDBM/13
  DO13/1 -> HEXDBM/14
  DO2/1 -> HEXDBM/3
  DO3_PWM/1 -> BITOP/1, HEXDBM/4
  DO4/1 -> HEXDBM/5
  DO5_PWM/1 -> BITOP_1/1, HEXDBM/6
  DO6_PWM/1 -> BITOP_2/1, HEXDBM/7
  DO7/1 -> HEXDBM/8
  DO8/1 -> HEXDBM/9
  DO9_PWM/1 -> BITOP_3/1, HEXDBM/10
  DO_A0/1 -> HEXDBM/15
  DO_A1/1 -> HEXDBM/16
  DO_A2/1 -> OCTBM/1
  DO_A3/1 -> OCTBM/2
  DO_A4/1 -> OCTBM/3
  DO_A5/1 -> OCTBM/4
  ERR_demux/1(err_code) -> err_code/1
  ERR_demux/2(err_subcode) -> err_subcode/1
  ERR_demux/3(status) -> comm_status/1
  HEXDBD/3 -> DI2/1
  HEXDBD/4 -> DI3/1
  HEXDBD/5 -> DI4/1
  HEXDBD/6 -> DI5/1
  HEXDBD/7 -> DI6/1
  HEXDBD/8 -> DI7/1
  HEXDBD/9 -> DI8/1
  HEXDBD/10 -> DI9/1
  HEXDBD/11 -> DI10/1
  HEXDBD/12 -> DI11/1
  HEXDBD/13 -> DI1/1
  HEXDBD/14 -> DI12/1
  HEXDBD/15 -> DI_A0/1
  HEXDBD/16 -> DI_A1/1
  HEXDBM/1 -> BITOP_10/1
  ISSW/1 -> REXLANG_REXduino/13
  MP_FORCE_RECONNECT/1 -> OCTBM_DEBUG/1
  MP_LOG_MASTER_VERSION/1 -> OCTBM_DEBUG/5
  MP_LOG_PINMODES/1 -> OCTBM_DEBUG/2
  OCTBD/1 -> DI_A2/1
  OCTBD/2 -> DI_A3/1
  OCTBD/3 -> DI_A4/1
  OCTBD/4 -> DI_A5/1
  OCTBM/1 -> BITOP_10/2
  OCTBM_DEBUG/1 -> REXLANG_REXduino/16
  REXLANG_REXduino/2 -> HEXDBD/1, OCTBD/1
  REXLANG_REXduino/3 -> AI_demux1/1(AI_data)
  REXLANG_REXduino/4 -> AI_demux2/1(AI_data)
  REXLANG_REXduino/5 -> OW_2_3_data/1
  REXLANG_REXduino/6 -> OW_4_5_data/1
  REXLANG_REXduino/7 -> OW_6_7_data/1
  REXLANG_REXduino/8 -> CNT2/1
  REXLANG_REXduino/9 -> CNT3/1
  REXLANG_REXduino/10 -> ERR_demux/1(data)
  REXLANG_REXduino/11 -> OW_8_9_data/1
  REXLANG_REXduino/12 -> OW_10_11_data/1
  REXLANG_REXduino/13 -> OW_12_data/1
  REXLANG_REXduino/14 -> OW_A0_A1_data/1
  REXLANG_REXduino/15 -> OW_A2_A3_data/1
  REXLANG_REXduino/16 -> OW_A4_A5_data/1
  REXLANG_REXduino/17 -> userRecv/1
  Simulation_Detector/1(Y) -> ISSW/3
  userSend/1 -> REXLANG_REXduino/18

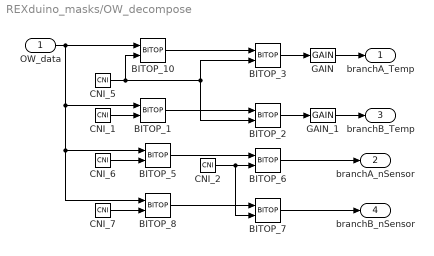
== system REXduino_masks/OW_decompose ==
  OW_data : Inport  Port=1  PortWidth=-1  SampleTime=-1  DataType=auto
      settings: SignalType=auto
  BITOP_1 : logiclib/BITOP  iop=5: Shift Left
  BITOP_10 : logiclib/BITOP  iop=5: Shift Left
  BITOP_{2..3,5,8} (4 alike) : logiclib/BITOP  iop=6: Shift Right
  BITOP_6 : logiclib/BITOP  iop=3: Bit AND
  BITOP_7 : logiclib/BITOP  iop=3: Bit AND
  CNI_1 : mathlib/CNI  icn=4
  CNI_2 : mathlib/CNI  icn=15
  CNI_5 : mathlib/CNI  icn=20
  CNI_6 : mathlib/CNI  icn=12
  CNI_7 : mathlib/CNI  icn=28
  GAIN : mathlib/GAIN  k=0.0625
  GAIN_1 : mathlib/GAIN  k=0.0625
  branchA_Temp : Outport  Port=1
  branchA_nSensor : Outport  Port=2
  branchB_Temp : Outport  Port=3
  branchB_nSensor : Outport  Port=4
  wires:
  BITOP_1/1 -> BITOP_2/1
  BITOP_10/1 -> BITOP_3/1
  BITOP_2/1 -> GAIN_1/1
  BITOP_3/1 -> GAIN/1
  BITOP_5/1 -> BITOP_6/1
  BITOP_6/1 -> branchA_nSensor/1
  BITOP_7/1 -> branchB_nSensor/1
  BITOP_8/1 -> BITOP_7/1
  CNI_1/1 -> BITOP_1/2
  CNI_2/1 -> BITOP_6/2, BITOP_7/2
  CNI_5/1 -> BITOP_10/2, BITOP_2/2, BITOP_3/2
  CNI_6/1 -> BITOP_5/2
  CNI_7/1 -> BITOP_8/2
  GAIN/1 -> branchA_Temp/1
  GAIN_1/1 -> branchB_Temp/1
  OW_data/1 -> BITOP_10/1, BITOP_1/1, BITOP_5/1, BITOP_8/1

== system REXduino_masks/OW_sensors_13_15 ==
  Temp : Inport  Port=1  PortWidth=-1  SampleTime=-1  DataType=auto
      settings: SignalType=auto
  nSensor : Inport  Port=2  PortWidth=-1  SampleTime=-1  DataType=auto
      settings: SignalType=auto
  ITOI_1 : logiclib/ITOI  BINF=off  fktab=[0 0 0 0 0 0 0 0 0 0 0 0 1 2 4]
  SHLD1 : analoglib/SHLD  y0=0  mode=1: Triggered sampling
  SHLD2 : analoglib/SHLD  y0=0  mode=1: Triggered sampling
  SHLD3 : analoglib/SHLD  y0=0  mode=1: Triggered sampling
  Sensor13 : Outport  Port=1
  Sensor14 : Outport  Port=2
  Sensor15 : Outport  Port=3
  wires:
  ITOI_1/2 -> SHLD1/2
  ITOI_1/3 -> SHLD2/2
  ITOI_1/4 -> SHLD3/2
  SHLD1/1 -> Sensor13/1
  SHLD2/1 -> Sensor14/1
  SHLD3/1 -> Sensor15/1
  Temp/1 -> SHLD2/1, SHLD3/1, SHLD1/1
  nSensor/1 -> ITOI_1/1

== system REXduino_masks/OW_sensors_1_4 ==
  Temp : Inport  Port=1  PortWidth=-1  SampleTime=-1  DataType=auto
      settings: SignalType=auto
  nSensor : Inport  Port=2  PortWidth=-1  SampleTime=-1  DataType=auto
      settings: SignalType=auto
  ITOI_1 : logiclib/ITOI  BINF=off  fktab=[0 1 2 4 8 0 0 0 0 0 0 0 0 0 0 0]
  SHLD{1..4} (4 alike) : analoglib/SHLD  y0=0  mode=1: Triggered sampling
  Sensor1 : Outport  Port=1
  Sensor2 : Outport  Port=2
  Sensor3 : Outport  Port=3
  Sensor4 : Outport  Port=4
  wires:
  ITOI_1/2 -> SHLD1/2
  ITOI_1/3 -> SHLD2/2
  ITOI_1/4 -> SHLD3/2
  ITOI_1/5 -> SHLD4/2
  SHLD1/1 -> Sensor1/1
  SHLD2/1 -> Sensor2/1
  SHLD3/1 -> Sensor3/1
  SHLD4/1 -> Sensor4/1
  Temp/1 -> SHLD3/1, SHLD4/1, SHLD2/1, SHLD1/1
  nSensor/1 -> ITOI_1/1

== system REXduino_masks/OW_sensors_5_8 ==
  Temp : Inport  Port=1  PortWidth=-1  SampleTime=-1  DataType=auto
      settings: SignalType=auto
  nSensor : Inport  Port=2  PortWidth=-1  SampleTime=-1  DataType=auto
      settings: SignalType=auto
  ITOI_1 : logiclib/ITOI  BINF=off  fktab=[0 1 2 4 8 0 0 0 0 0 0 0 0 0 0 0]
  SHLD{1..4} (4 alike) : analoglib/SHLD  y0=0  mode=1: Triggered sampling
  Sensor5 : Outport  Port=1
  Sensor6 : Outport  Port=2
  Sensor7 : Outport  Port=3
  Sensor8 : Outport  Port=4
  wires:
  ITOI_1/2 -> SHLD1/2
  ITOI_1/3 -> SHLD2/2
  ITOI_1/4 -> SHLD3/2
  ITOI_1/5 -> SHLD4/2
  SHLD1/1 -> Sensor5/1
  SHLD2/1 -> Sensor6/1
  SHLD3/1 -> Sensor7/1
  SHLD4/1 -> Sensor8/1
  Temp/1 -> SHLD3/1, SHLD4/1, SHLD2/1, SHLD1/1
  nSensor/1 -> ITOI_1/1

== system REXduino_masks/OW_sensors_9_12 ==
  Temp : Inport  Port=1  PortWidth=-1  SampleTime=-1  DataType=auto
      settings: SignalType=auto
  nSensor : Inport  Port=2  PortWidth=-1  SampleTime=-1  DataType=auto
      settings: SignalType=auto
  ITOI_1 : logiclib/ITOI  BINF=off  fktab=[0 0 0 0 0 0 0 0 0 1 2 4 8 0 0 0]
  SHLD{1..4} (4 alike) : analoglib/SHLD  y0=0  mode=1: Triggered sampling
  Sensor9 : Outport  Port=1
  Sensor10 : Outport  Port=2
  Sensor11 : Outport  Port=3
  Sensor12 : Outport  Port=4
  wires:
  ITOI_1/2 -> SHLD1/2
  ITOI_1/3 -> SHLD2/2
  ITOI_1/4 -> SHLD3/2
  ITOI_1/5 -> SHLD4/2
  SHLD1/1 -> Sensor9/1
  SHLD2/1 -> Sensor10/1
  SHLD3/1 -> Sensor11/1
  SHLD4/1 -> Sensor12/1
  Temp/1 -> SHLD3/1, SHLD4/1, SHLD2/1, SHLD1/1
  nSensor/1 -> ITOI_1/1

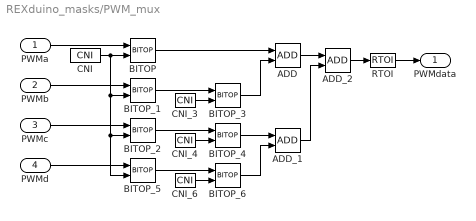
== system REXduino_masks/PWM_mux ==
  PWMa : Inport  Port=1  PortWidth=-1  SampleTime=-1  DataType=auto
      settings: SignalType=auto
  PWMb : Inport  Port=2  PortWidth=-1  SampleTime=-1  DataType=auto
      settings: SignalType=auto
  PWMc : Inport  Port=3  PortWidth=-1  SampleTime=-1  DataType=auto
      settings: SignalType=auto
  PWMd : Inport  Port=4  PortWidth=-1  SampleTime=-1  DataType=auto
      settings: SignalType=auto
  ADD : mathlib/ADD
  ADD_1 : mathlib/ADD
  ADD_2 : mathlib/ADD
  BITOP : logiclib/BITOP  iop=3: Bit AND
  BITOP_1 : logiclib/BITOP  iop=3: Bit AND
  BITOP_2 : logiclib/BITOP  iop=3: Bit AND
  BITOP_3 : logiclib/BITOP  iop=5: Shift Left
  BITOP_4 : logiclib/BITOP  iop=5: Shift Left
  BITOP_5 : logiclib/BITOP  iop=3: Bit AND
  BITOP_6 : logiclib/BITOP  iop=5: Shift Left
  CNI : mathlib/CNI  icn=255
  CNI_3 : mathlib/CNI  icn=8
  CNI_4 : mathlib/CNI  icn=16
  CNI_6 : mathlib/CNI  icn=24
  RTOI : mathlib/RTOI
  PWMdata : Outport  Port=1
  wires:
  ADD/1 -> ADD_2/1
  ADD_1/1 -> ADD_2/2
  ADD_2/1 -> RTOI/1
  BITOP/1 -> ADD/1
  BITOP_1/1 -> BITOP_3/1
  BITOP_2/1 -> BITOP_4/1
  BITOP_3/1 -> ADD/2
  BITOP_4/1 -> ADD_1/1
  BITOP_5/1 -> BITOP_6/1
  BITOP_6/1 -> ADD_1/2
  CNI/1 -> BITOP/2, BITOP_1/2, BITOP_2/2, BITOP_5/2
  CNI_3/1 -> BITOP_3/2
  CNI_4/1 -> BITOP_4/2
  CNI_6/1 -> BITOP_6/2
  PWMa/1 -> BITOP/1
  PWMb/1 -> BITOP_1/1
  PWMc/1 -> BITOP_2/1
  PWMd/1 -> BITOP_5/1
  RTOI/1 -> PWMdata/1

== system REXduino_masks/Arduino_MEGA2560/AI_demux1 ==
  AI_data : Inport  Port=1  PortWidth=-1  SampleTime=-1  DataType=auto
      settings: SignalType=auto
  BITOP_1 : logiclib/BITOP  iop=6: Shift Right
  BITOP_10 : logiclib/BITOP  iop=3: Bit AND
  BITOP_2 : logiclib/BITOP  iop=3: Bit AND
  BITOP_3 : logiclib/BITOP  iop=6: Shift Right
  BITOP_4 : logiclib/BITOP  iop=3: Bit AND
  CNI : mathlib/CNI  icn=1023
  CNI_1 : mathlib/CNI  icn=10
  AIdata1 : Outport  Port=1
  AIdata2 : Outport  Port=2
  AIdata3 : Outport  Port=3
  wires:
  AI_data/1 -> BITOP_1/1, BITOP_10/1
  BITOP_1/1 -> BITOP_2/1, BITOP_3/1
  BITOP_10/1 -> AIdata1/1
  BITOP_2/1 -> AIdata2/1
  BITOP_3/1 -> BITOP_4/1
  BITOP_4/1 -> AIdata3/1
  CNI/1 -> BITOP_10/2, BITOP_2/2, BITOP_4/2
  CNI_1/1 -> BITOP_1/2, BITOP_3/2

== system REXduino_masks/Arduino_MEGA2560/AI_demux2 ==
  AI_data : Inport  Port=1  PortWidth=-1  SampleTime=-1  DataType=auto
      settings: SignalType=auto
  BITOP_1 : logiclib/BITOP  iop=6: Shift Right
  BITOP_10 : logiclib/BITOP  iop=3: Bit AND
  BITOP_2 : logiclib/BITOP  iop=3: Bit AND
  BITOP_3 : logiclib/BITOP  iop=6: Shift Right
  BITOP_4 : logiclib/BITOP  iop=3: Bit AND
  CNI : mathlib/CNI  icn=1023
  CNI_1 : mathlib/CNI  icn=10
  AIdata1 : Outport  Port=1
  AIdata2 : Outport  Port=2
  AIdata3 : Outport  Port=3
  wires:
  AI_data/1 -> BITOP_1/1, BITOP_10/1
  BITOP_1/1 -> BITOP_2/1, BITOP_3/1
  BITOP_10/1 -> AIdata1/1
  BITOP_2/1 -> AIdata2/1
  BITOP_3/1 -> BITOP_4/1
  BITOP_4/1 -> AIdata3/1
  CNI/1 -> BITOP_10/2, BITOP_2/2, BITOP_4/2
  CNI_1/1 -> BITOP_1/2, BITOP_3/2

== system REXduino_masks/Arduino_MEGA2560/AI_demux3 ==
  AI_data : Inport  Port=1  PortWidth=-1  SampleTime=-1  DataType=auto
      settings: SignalType=auto
  BITOP_1 : logiclib/BITOP  iop=6: Shift Right
  BITOP_10 : logiclib/BITOP  iop=3: Bit AND
  BITOP_2 : logiclib/BITOP  iop=3: Bit AND
  BITOP_3 : logiclib/BITOP  iop=6: Shift Right
  BITOP_4 : logiclib/BITOP  iop=3: Bit AND
  CNI : mathlib/CNI  icn=1023
  CNI_1 : mathlib/CNI  icn=10
  AIdata1 : Outport  Port=1
  AIdata2 : Outport  Port=2
  AIdata3 : Outport  Port=3
  wires:
  AI_data/1 -> BITOP_1/1, BITOP_10/1
  BITOP_1/1 -> BITOP_2/1, BITOP_3/1
  BITOP_10/1 -> AIdata1/1
  BITOP_2/1 -> AIdata2/1
  BITOP_3/1 -> BITOP_4/1
  BITOP_4/1 -> AIdata3/1
  CNI/1 -> BITOP_2/2, BITOP_4/2, BITOP_10/2
  CNI_1/1 -> BITOP_1/2, BITOP_3/2

== system REXduino_masks/Arduino_MEGA2560/CNT_mux ==
  CNT2R : Inport  Port=1  PortWidth=-1  SampleTime=-1  DataType=auto
      settings: SignalType=auto
  CNT2E : Inport  Port=2  PortWidth=-1  SampleTime=-1  DataType=auto
      settings: SignalType=auto
  CNT3R : Inport  Port=3  PortWidth=-1  SampleTime=-1  DataType=auto
      settings: SignalType=auto
  CNT3E : Inport  Port=4  PortWidth=-1  SampleTime=-1  DataType=auto
      settings: SignalType=auto
  OCTBM : logiclib/BMOCT  shift=0
  cntCmd : Outport  Port=1
  wires:
  CNT2E/1 -> OCTBM/2
  CNT2R/1 -> OCTBM/1
  CNT3E/1 -> OCTBM/4
  CNT3R/1 -> OCTBM/3
  OCTBM/1 -> cntCmd/1
